simulink model "Punto4"  (R2024b)
settings: Solver=VariableStepAuto  StartTime=0.0  StopTime=50  RelTol=1e-3
libraries: simulink x2
settings Model: Creator=Andres Felipe  LastModifiedBy=Andres Felipe

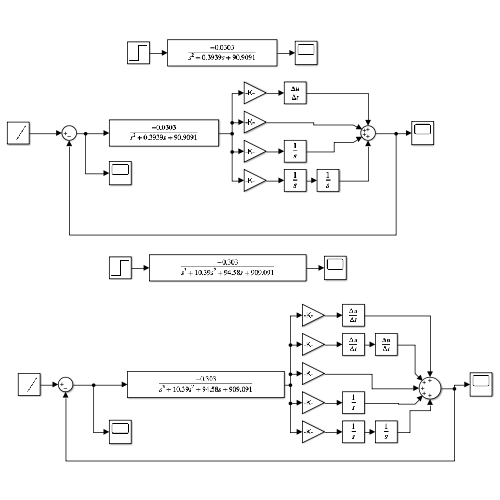
[thumbnail: Simulink's stored preview of the top-level diagram]
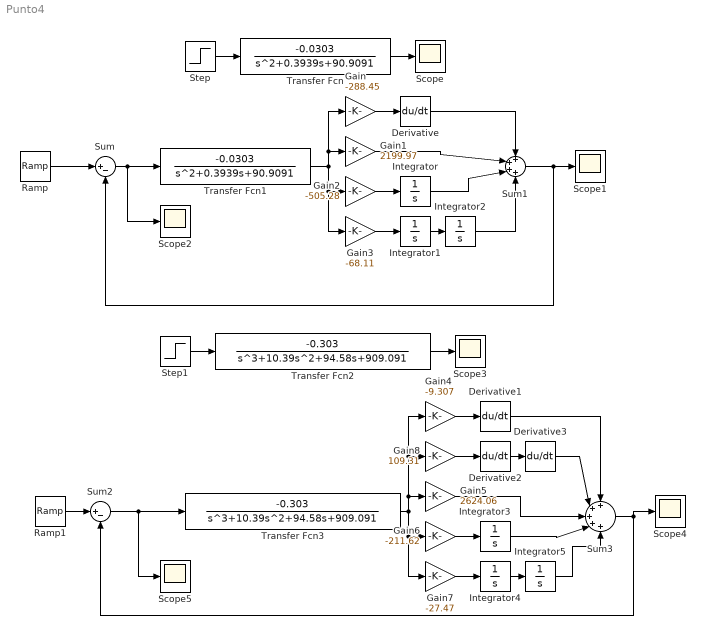
== system Punto4 ==
  Derivative{,1..3} (4 alike) : Derivative
  Gain : Gain  Gain=-288.45
  Gain1 : Gain  Gain=2199.97
  Gain2 : Gain  Gain=-505.28
  Gain3 : Gain  Gain=-68.11
  Gain4 : Gain  Gain=-9.307
  Gain5 : Gain  Gain=2624.06
  Gain6 : Gain  Gain=-211.62
  Gain7 : Gain  Gain=-27.47
  Gain8 : Gain  Gain=109.31
  Integrator{,1..5} (6 alike) : Integrator
  Ramp : simulink/Sources/Ramp  slope=1  start=0  InitialOutput=0
  Ramp1 : simulink/Sources/Ramp  slope=1  start=0  InitialOutput=0
  Scope{,1..5} (6 alike) : Scope
  Step : Step  Time=0  SampleTime=0
  Step1 : Step  Time=0  SampleTime=0
  Sum : Sum  Inputs=|+-
  Sum1 : Sum  Inputs=++++
  Sum2 : Sum  Inputs=|+-
  Sum3 : Sum  Inputs=+++++
  Transfer Fcn : TransferFcn  Numerator=[-0.0303]  Denominator=[1 0.3939 90.9091]
  Transfer Fcn1 : TransferFcn  Numerator=[-0.0303]  Denominator=[1 0.3939 90.9091]
  Transfer Fcn2 : TransferFcn  Numerator=[-0.303]  Denominator=[1 10.39 94.58 909.091]
  Transfer Fcn3 : TransferFcn  Numerator=[-0.303]  Denominator=[1 10.39 94.58 909.091]
  wires:
  Step/1 -> Transfer Fcn/1
  Transfer Fcn/1 -> Scope/1
  Sum/1 -> Scope2/1, Transfer Fcn1/1
  Sum1/1 -> Sum/2, Scope1/1
  Ramp/1 -> Sum/1
  Gain/1 -> Derivative/1
  Gain2/1 -> Integrator/1
  Gain3/1 -> Integrator1/1
  Integrator1/1 -> Integrator2/1
  Derivative/1 -> Sum1/1
  Gain1/1 -> Sum1/2
  Integrator/1 -> Sum1/3
  Integrator2/1 -> Sum1/4
  Transfer Fcn1/1 -> Gain3/1, Gain2/1, Gain/1, Gain1/1
  Transfer Fcn2/1 -> Scope3/1
  Step1/1 -> Transfer Fcn2/1
  Transfer Fcn3/1 -> Gain4/1, Gain8/1, Gain5/1, Gain7/1, Gain6/1
  Gain6/1 -> Integrator3/1
  Gain4/1 -> Derivative1/1
  Gain7/1 -> Integrator4/1
  Sum2/1 -> Scope5/1, Transfer Fcn3/1
  Integrator5/1 -> Sum3/5
  Integrator3/1 -> Sum3/4
  Sum3/1 -> Scope4/1, Sum2/2
  Integrator4/1 -> Integrator5/1
  Gain5/1 -> Sum3/3
  Ramp1/1 -> Sum2/1
  Derivative1/1 -> Sum3/1
  Gain8/1 -> Derivative2/1
  Derivative2/1 -> Derivative3/1
  Derivative3/1 -> Sum3/2
